simulink model "Q4PWM"  (R2013a)
settings: Solver=ode45  StartTime=0.0  StopTime=0.5  MaxStep=1e-4  RelTol=1e-3
libraries: simulink x1
settings Model: Creator=Sony  LastModifiedBy=Sony

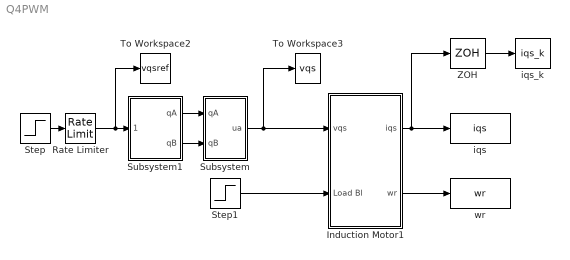
== system Q4PWM ==
  Induction Motor1 : Subsystem  mask{Rr=0.183, Rs=0.277, Ra=0.277+0.183*(0.0553/0.05606), Lr=0.05606, Ls=0.0553, Lm=0.0538, La=0.0553-((0.0538*0.0538)/0.05606), J=0.0165, B=0.025, ws=2*pi*60, P=4, ids=6, Km=36.224, Tm=0.33}
      mask prompts: Rr "Rr (ohm)"; Rs "Rs (ohm)"; Ra "Ra (ohm)"; Lr "Lr (H)"; Ls "Ls (H)"; Lm "Lm (H)"; La "La (H)"; J "J (kgm^2)"; B "B (kgm^2/s)"; ws "ws (rad/s)"; ids "ids (A)"
  Rate Limiter : RateLimiter  RisingSlewLimit=(200*sqrt(2)/sqrt(3))/0.1
  Step : Step  Time=0.1  After=200*sqrt(2)/sqrt(3)  SampleTime=0
  Step1 : Step  Time=0.3  After=0.025  SampleTime=0
  Subsystem : Subsystem  mask{Udc=170}
  Subsystem1 : Subsystem  mask{Udc=170, Tsw=1e-5}
  To Workspace2 : ToWorkspace  VariableName=vqsref  SampleTime=-1  SaveFormat=Timeseries
  To Workspace3 : ToWorkspace  VariableName=vqs  SampleTime=-1  SaveFormat=Timeseries
  ZOH : ZeroOrderHold  SampleTime=(200e-6)/2
  iqs : ToWorkspace  VariableName=iqs  SampleTime=-1  SaveFormat=Timeseries
  iqs_k : ToWorkspace  VariableName=iqs_k  SampleTime=-1  SaveFormat=Timeseries
  wr : ToWorkspace  VariableName=wr  SampleTime=-1  SaveFormat=Timeseries
  wires:
  Induction Motor1/2(wr) -> wr/1
  Step/1 -> Rate Limiter/1
  Step1/1 -> Induction Motor1/2(Load Bl)
  Induction Motor1/1(iqs) -> ZOH/1, iqs/1
  Rate Limiter/1 -> Subsystem1/1(vqsref), To Workspace2/1
  ZOH/1 -> iqs_k/1
  Subsystem/1(ua) -> Induction Motor1/1(vqs), To Workspace3/1
  Subsystem1/1(qA) -> Subsystem/1(qA)
  Subsystem1/2(qB) -> Subsystem/2(qB)

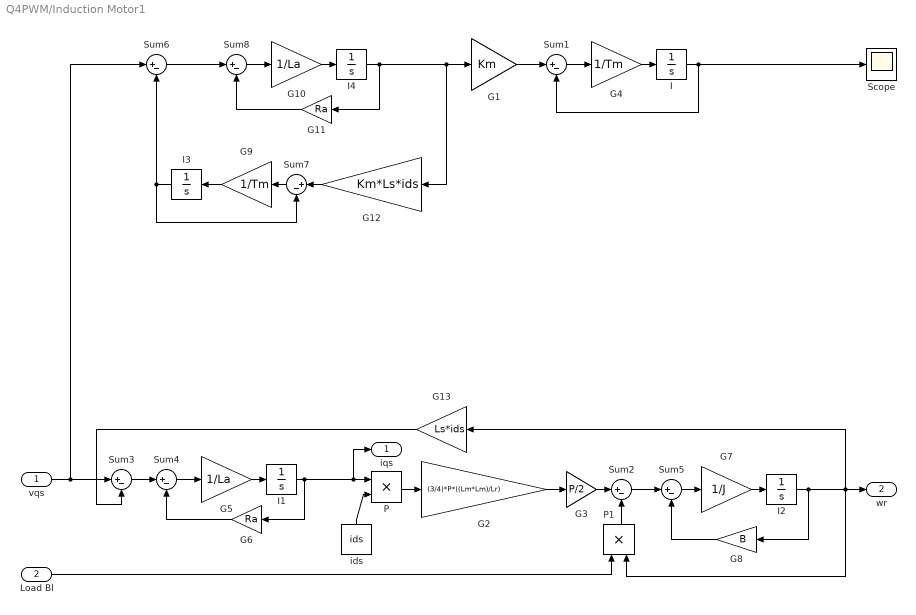
== system Q4PWM/Induction Motor1 ==
  vqs : Inport
  Load Bl : Inport  Port=2
  G1 : Gain  Gain=Km
  G10 : Gain  Gain=1/La
  G11 : Gain  Gain=Ra
  G12 : Gain  Gain=Km*Ls*ids
  G13 : Gain  Gain=Ls*ids
  G2 : Gain  Gain=(3/4)*P*((Lm*Lm)/Lr)
  G3 : Gain  Gain=P/2
  G4 : Gain  Gain=1/Tm
  G5 : Gain  Gain=1/La
  G6 : Gain  Gain=Ra
  G7 : Gain  Gain=1/J
  G8 : Gain  Gain=B
  G9 : Gain  Gain=1/Tm
  I{,1..4} (5 alike) : Integrator
  P : Product
  P1 : Product
  Scope : Scope
  Sum{1..8} (8 alike) : Sum  Inputs=|+-
  ids : Constant  Value=ids
  iqs : Outport
  wr : Outport  Port=2
  wires:
  vqs/1 -> Sum6/1, Sum3/1
  I1/1 -> P/1, iqs/1, G6/1
  P/1 -> G2/1
  Load Bl/1 -> P1/1
  G2/1 -> G3/1
  G3/1 -> Sum2/1
  P1/1 -> Sum2/2
  Sum2/1 -> Sum5/1
  G13/1 -> Sum3/2
  I2/1 -> G8/1, G13/1, P1/2, wr/1
  I/1 -> Sum1/2, Scope/1
  Sum1/1 -> G4/1
  G4/1 -> I/1
  G1/1 -> Sum1/1
  G6/1 -> Sum4/2
  Sum4/1 -> G5/1
  G5/1 -> I1/1
  Sum3/1 -> Sum4/1
  G8/1 -> Sum5/2
  Sum5/1 -> G7/1
  G7/1 -> I2/1
  I3/1 -> Sum6/2, Sum7/2
  Sum7/1 -> G9/1
  G9/1 -> I3/1
  G12/1 -> Sum7/1
  I4/1 -> G12/1, G1/1, G11/1
  G11/1 -> Sum8/2
  Sum8/1 -> G10/1
  G10/1 -> I4/1
  Sum6/1 -> Sum8/1
  ids/1 -> P/2

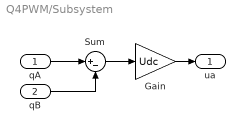
== system Q4PWM/Subsystem ==
  qA : Inport
  qB : Inport  Port=2
  Gain : Gain  Gain=Udc
  Sum : Sum  Inputs=|+-
  ua : Outport
  wires:
  qA/1 -> Sum/1
  Sum/1 -> Gain/1
  qB/1 -> Sum/2
  Gain/1 -> ua/1

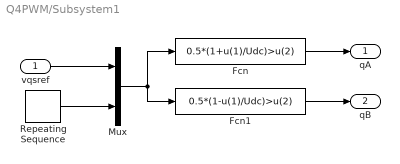
== system Q4PWM/Subsystem1 ==
  vqsref : Inport
  Fcn : Fcn  Expr=0.5*(1+u(1)/Udc)>u(2)
  Fcn1 : Fcn  Expr=0.5*(1-u(1)/Udc)>u(2)
  Mux : Mux  Inputs=2
  Repeating Sequence : simulink/Sources/Repeating Sequence  rep_seq_t=Tsw*[0 0.5 1]  rep_seq_y=[1 0 1]
  qA : Outport
  qB : Outport  Port=2
  wires:
  Repeating Sequence/1 -> Mux/2
  Mux/1 -> Fcn/1, Fcn1/1
  vqsref/1 -> Mux/1
  Fcn/1 -> qA/1
  Fcn1/1 -> qB/1
